simulink model "stateflow_daigram"  (R2020a)
settings: Solver=FixedStepDiscrete  StartTime=0.0  StopTime=10.0  FixedStep=0.1  RelTol=1e-3  EnableMultiTasking=on
settings Model: Creator=91968  LastModifiedBy=91968
settings SolverCC: AutoInsertRateTranBlk=on
settings DataIOCC: LimitDataPoints=on
settings OptimizationCC: LifeSpan=inf
settings DebuggingCC: AllowSymbolicDim=off  SFUnexpectedBacktrackingDiag=warning  SFNoUnconditionalDefaultTransitionDiag=warning  SFExecutionAtInitializationDiag=none  ArithmeticOperatorsInVariantConditions=warning
settings SFSimCC: SimUseLocalCustomCode=off  CustomCodeUndefinedFunction=UseInterfaceOnly
settings RTWCC: RTWUseLocalCustomCode=off
settings CodeAppCC: StateflowObjectComments=on
settings GRTTargetCC: TargetLangStandard=C89/C90 (ANSI)
settings ConfigComp: CovMetricSettings=dw  CovHtmlReporting=on  CovSaveCumulativeToWorkspaceVar=on  CovSaveSingleToWorkspaceVar=on  CovShowResultsExplorer=off  CovExternalEMLEnable=off

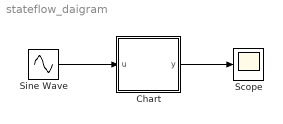
== system stateflow_daigram ==
  Chart : Stateflow chart  TreatAsAtomicUnit=on
  Scope : Scope
  Sine Wave : Sin  SampleTime=0
  wires:
  Sine Wave/1 -> Chart/1(u)
  Chart/1(y) -> Scope/1

== stateflow chart stateflow_daigram/Chart ==
  state ACC_OFF_MODE
    entry:
    Acceleration_Mode = 0;
  state ACC_STANDBY_MODE
    entry:
    Acceleration_Mode = 1;
  state ACC_ON_MODE
    state LeadVehicle_Detected_Default
      entry:
      Acceleration_Mode= 2;
    state LeadVehicle_Not_Detected
      entry:
      Acceleration_Mode= 1;
    (default) -> LeadVehicle_Not_Detected
    LeadVehicle_Not_Detected -> LeadVehicle_Detected_Default : [(LeadVehicle_Detected==1) && ...
        | (DriveVehicleSpeed == SetSpeed)]
    LeadVehicle_Detected_Default -> LeadVehicle_Not_Detected : [LeadVehicle_Detected == 0]
  (default) -> ACC_OFF_MODE
  ACC_OFF_MODE -> ACC_STANDBY_MODE : [CruiseSwitch == 1]
  ACC_STANDBY_MODE -> ACC_OFF_MODE [order 1] : [CruiseSwitch==0]
  ACC_ON_MODE -> ACC_STANDBY_MODE [order 2] : [SetSwitch ==0]
  ACC_STANDBY_MODE -> ACC_ON_MODE [order 2] : [SetSwitch ==1]
  ACC_ON_MODE -> ACC_OFF_MODE [order 1] : [CruiseSwitch == 0]
  data: u input; y output
